simulink model "aerodymic_modules"  (R2023b)
settings: Solver=VariableStepAuto  StartTime=0.0  StopTime=simtime  MaxStep=0.00005  RelTol=1e-3
undefined symbols (not defined in the file): c_aero, c_drt, dpomega0, dpomega1, dpv1, dpv2, H_gen, H_WTR, k_a, k_aero, k_drt, lambda_opt, omega_0, omega_WTR_0, omega_WTR_n, p_avail, p_init, R_WTR, tau_init, Theta_0, Theta_vw2, Theta_w0, v_omega_1, v_w_0, v_w_min, v_w_n
settings Model: Creator=s183702  LastModifiedBy=marti

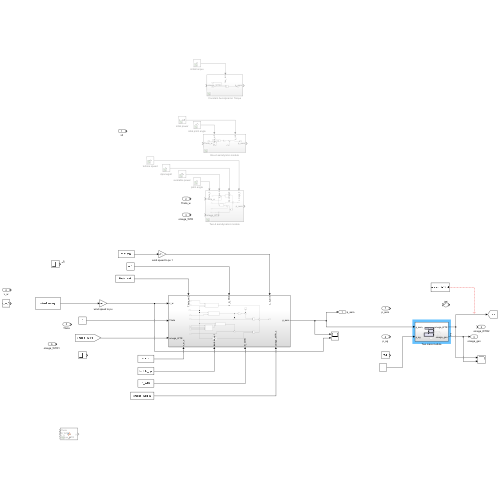
[thumbnail: Simulink's stored preview of the top-level diagram]
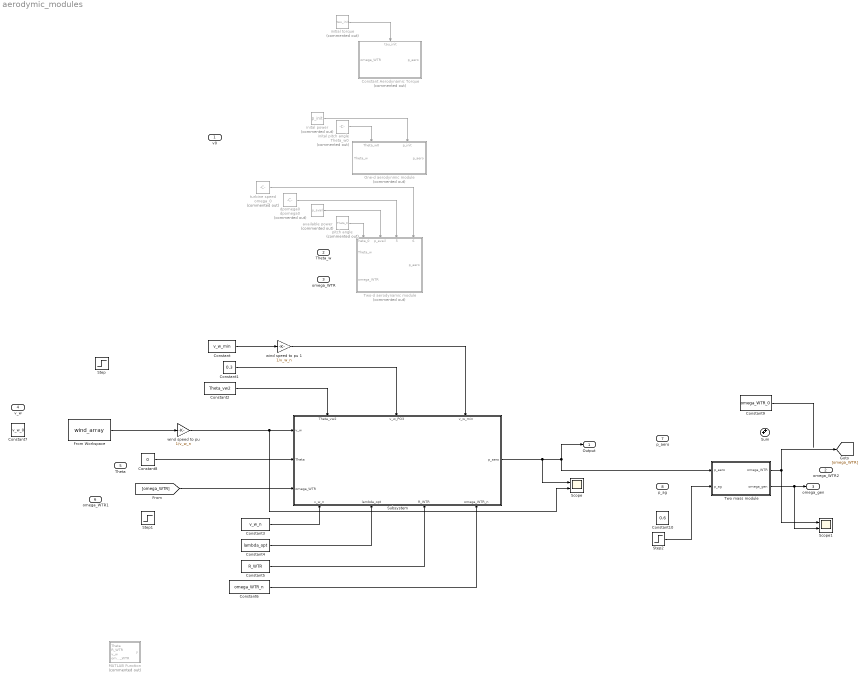
== system aerodymic_modules ==
  v0 : Inport
  Theta_w : Inport  Port=2
  omega_WTR : Inport  Port=3
  v_w : Inport  Port=4
  Theta : Inport  Port=5
  omega_WTR1 : Inport  Port=6
  p_aero : Inport  Port=7
  p_ag : Inport  Port=8
  Constant : Constant  Value=v_w_min
  Constant Aerodynamic Torque : Subsystem  Commented=on
      settings: PortSchema="{\"entries\":[{\"content\":{\"sides\":[{\"content\":{\"connectorIds\":[\"In1\"]},\"type\":\"ConnectorPlacement.EquallySpacedRectSide\",\"uuid\":\"8856b20c-a913-4b1f-bb06-3bfd5591729e\"},{\"content\":{\"connectorIds\":[\"Out1\"],\"side\":\"RIGHT\"},\"type\":\"ConnectorPlacement.EquallySpacedRectSide\",\"uuid\":\"d2cddd21-94c4-4346-9f93-c8cf69895e41\"},{\"content\":{\"connectorIds\":[\"In2\"],\"side\":\"TOP\"},\"type\":\"ConnectorPlacement.EquallySpacedRectSide\",\"uuid\":\"bedbe1d1-3c36-4165-aa7e-0fef857489e1\"},{\"content\":{\"side\":\"BOTTOM\"},\"type\":\"ConnectorPlacement.EquallySpacedRectSide\",\"uuid\":\"8fbc4b09-9296-41c8-ae54-d2fa1c44f1b6\"}]},\"type\":\"ConnectorPlacement.EquallySpacedConnector\",\"uuid\":\"9cd9660b-1bf9-4aa1-9147-9c9a71ae45e0\"}],\"packageUris\":[\"http://schema.mathworks.com/mf0/Connector/R2020b\"],\"version\":\"1.0\"}"
  Constant1 : Constant  Value=0.3
  Constant10 : Constant  Value=0.6
  Constant2 : Constant  Value=Theta_vw2
  Constant3 : Constant  Value=v_w_n
  Constant4 : Constant  Value=lambda_opt
  Constant5 : Constant  Value=R_WTR
  Constant6 : Constant  Value=omega_WTR_n
  Constant7 : Constant  Value=v_w_0
  Constant8 : Constant  Value=0
  Constant9 : Constant  Value=omega_WTR_0
  From Workspace : FromWorkspace  VariableName=wind_array
  MATLAB Function : MATLAB Function  Commented=on  TreatAsAtomicUnit=on
  One-d aerodynmic module : Subsystem  Commented=on
      settings: PortSchema="{\"entries\":[{\"content\":{\"sides\":[{\"content\":{\"connectorIds\":[\"In1\"]},\"type\":\"ConnectorPlacement.EquallySpacedRectSide\",\"uuid\":\"289bff7f-e2b1-4f4a-a280-3eccfab6ccfb\"},{\"content\":{\"connectorIds\":[\"Out1\"],\"side\":\"RIGHT\"},\"type\":\"ConnectorPlacement.EquallySpacedRectSide\",\"uuid\":\"ad352476-6e1f-4395-a3cf-73973636468c\"},{\"content\":{\"connectorIds\":[\"In2\",\"In3\"],\"side\":\"TOP\"},\"type\":\"ConnectorPlacement.EquallySpacedRectSide\",\"uuid\":\"0dc03381-ab12-4ca7-95d7-b6e9390f3624\"},{\"content\":{\"side\":\"BOTTOM\"},\"type\":\"ConnectorPlacement.EquallySpacedRectSide\",\"uuid\":\"0b978398-81f6-4235-820d-3640bddfbdb8\"}]},\"type\":\"ConnectorPlacement.EquallySpacedConnector\",\"uuid\":\"cacb7d17-2ea4-44c7-b4a3-963f0a31b934\"}],\"packageUris\":[\"http://schema.mathworks.com/mf0/Connector/R2020b\"],\"version\":\"1.0\"}"
  Scope : Scope  NumInputPorts=2
  Scope1 : Scope  NumInputPorts=2
  Step : Step  Time=11  Before=v_w_0  After=v_w_0+0.05  SampleTime=0
  Step1 : Step  Time=8  Before=omega_WTR_0  After=omega_WTR_0+0.1  SampleTime=0
  Step2 : Step  Time=20  Before=0.6  After=0.6  SampleTime=0
  Subsystem : Subsystem
      settings: PortSchema="{\"entries\":[{\"content\":{\"sides\":[{\"content\":{\"connectorIds\":[\"In1\",\"In2\",\"In3\"]},\"type\":\"ConnectorPlacement.EquallySpacedRectSide\",\"uuid\":\"ae3b79f5-547b-4d10-abca-a0aa9cd2564f\"},{\"content\":{\"connectorIds\":[\"Out1\"],\"side\":\"RIGHT\"},\"type\":\"ConnectorPlacement.EquallySpacedRectSide\",\"uuid\":\"c3c2b3cb-a75a-4372-91a9-47eb1a58d54f\"},{\"content\":{\"connectorIds\":[\"In4\",\"In5\",\"In6\"],\"side\":\"TOP\"},\"type\":\"ConnectorPlacement.EquallySpacedRectSide\",\"uuid\":\"49d081fd-d1d3-413c-affe-c564a0af719c\"},{\"content\":{\"connectorIds\":[\"In7\",\"In8\",\"In9\",\"In10\"],\"side\":\"BOTTOM\"},\"type\":\"ConnectorPlacement.EquallySpacedRectSide\",\"uuid\":\"c00a81a2-52c7-4daf-8b0c-a778841ec5d6\"}]},\"type\":\"ConnectorPlacement.EquallySpacedConnector\",\"uuid\":\"220248d6-ce4a-4e11-ab43-1d105a3d9686\"}],\"packageUris\":[\"http://schema.mathworks.com/mf0/Connector/R2020b\"],\"version\":\"1.0\"}"
  Sum : Sum  Inputs=++|
  Two mass module : Subsystem
  Two-d aerodynamic module : Subsystem  Commented=on
      settings: PortSchema="{\"entries\":[{\"content\":{\"sides\":[{\"content\":{\"connectorIds\":[\"In1\",\"In2\"]},\"type\":\"ConnectorPlacement.EquallySpacedRectSide\",\"uuid\":\"29aafb7d-ac63-4bda-a4d9-7691da9bab26\"},{\"content\":{\"connectorIds\":[\"Out1\"],\"side\":\"RIGHT\"},\"type\":\"ConnectorPlacement.EquallySpacedRectSide\",\"uuid\":\"d2e3e6f1-e433-4ce8-a4cd-da131dd7b9aa\"},{\"content\":{\"connectorIds\":[\"In3\",\"In4\",\"In5\",\"In6\"],\"side\":\"TOP\"},\"type\":\"ConnectorPlacement.EquallySpacedRectSide\",\"uuid\":\"d4b21252-afd5-4f00-9115-123c5cb74ac3\"},{\"content\":{\"side\":\"BOTTOM\"},\"type\":\"ConnectorPlacement.EquallySpacedRectSide\",\"uuid\":\"8ed30fa1-595f-4836-a19a-9de8ec421887\"}]},\"type\":\"ConnectorPlacement.EquallySpacedConnector\",\"uuid\":\"9c06a76b-7ab3-4f8d-9ed4-36342eae06f9\"}],\"packageUris\":[\"http://schema.mathworks.com/mf0/Connector/R2020b\"],\"version\":\"1.0\"}"
  available power : Constant  Commented=on  Value=p_avail
  dpomega0 : Constant  Commented=on  Value=dpomega0
  inital pitch angle : Constant  Commented=on  Value=Theta_w0
  inital power : Constant  Commented=on  Value=p_init
  initial torque : Constant  Commented=on  Value=tau_init
  pitch angle : Constant  Commented=on  Value=Theta_0
  turbine speed : Constant  Commented=on  Value=omega_0
  "wind speed to pu " : Gain  Gain=1/v_w_n
  wind speed to pu 1 : Gain  Gain=1/v_w_n
  Output : Outport  SignalName=p_aero
  omega_WTR2 : Outport  Port=2
  omega_gen : Outport  Port=3
  wires:
  initial torque/1 -> Constant Aerodynamic Torque/2(tau_init)
  inital pitch angle/1 -> One-d aerodynmic module/2(Theta_w0)
  inital power/1 -> One-d aerodynmic module/3(p_init)
  pitch angle/1 -> Two-d aerodynamic module/3(Theta_0)
  available power/1 -> Two-d aerodynamic module/4(p_avail)
  dpomega0/1 -> Two-d aerodynamic module/5(dpomega0)
  turbine speed/1 -> Two-d aerodynamic module/6(omega_0)
  Constant/1 -> wind speed to pu 1/1
  Constant1/1 -> Subsystem/5(v_w_PO3)
  From Workspace/1 -> "wind speed to pu "/1
  Constant2/1 -> Subsystem/4(Theta_vw2)
  Constant8/1 -> Subsystem/2(Theta)
  Constant3/1 -> Subsystem/7(v_w_n)
  Constant4/1 -> Subsystem/8(lambda_opt)
  Constant5/1 -> Subsystem/9(R_WTR)
  Constant6/1 -> Subsystem/10(omega_WTR_n)
  [omega_WTR] -> Subsystem/3(omega_WTR)
  wind speed to pu 1/1 -> Subsystem/6(v_w_min)
  Subsystem/1(p_aero) -> Scope/1, Two mass module/1(p_aero), Output/1
  Step2/1 -> Two mass module/2(p_ag)
  Two mass module/2(omega_gen) -> Scope1/2, omega_gen/1
  Constant9/1 -> ?
  Two mass module/1(omega_WTR) -> [omega_WTR], Scope1/1
  "wind speed to pu "/1 -> Scope/2, Subsystem/1(v_w)

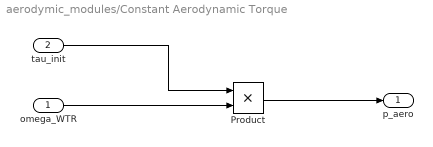
== system aerodymic_modules/Constant Aerodynamic Torque ==
  omega_WTR : Inport
  tau_init : Inport  Port=2
  Product : Product
  p_aero : Outport
  wires:
  omega_WTR/1 -> Product/2
  Product/1 -> p_aero/1
  tau_init/1 -> Product/1

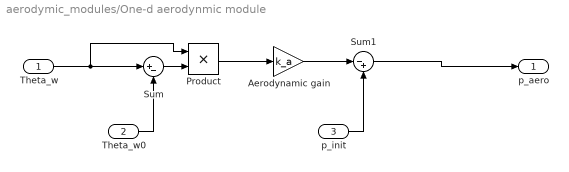
== system aerodymic_modules/One-d aerodynmic module ==
  Theta_w : Inport
  Theta_w0 : Inport  Port=2
  p_init : Inport  Port=3
  Aerodynamic gain : Gain  Gain=k_a
  Product : Product
  Sum : Sum  Inputs=|+-
  Sum1 : Sum  Inputs=|-+
  p_aero : Outport
  wires:
  Aerodynamic gain/1 -> Sum1/1
  Sum/1 -> Product/2
  Product/1 -> Aerodynamic gain/1
  Theta_w0/1 -> Sum/2
  p_init/1 -> Sum1/2
  Theta_w/1 -> Product/1, Sum/1
  Sum1/1 -> p_aero/1

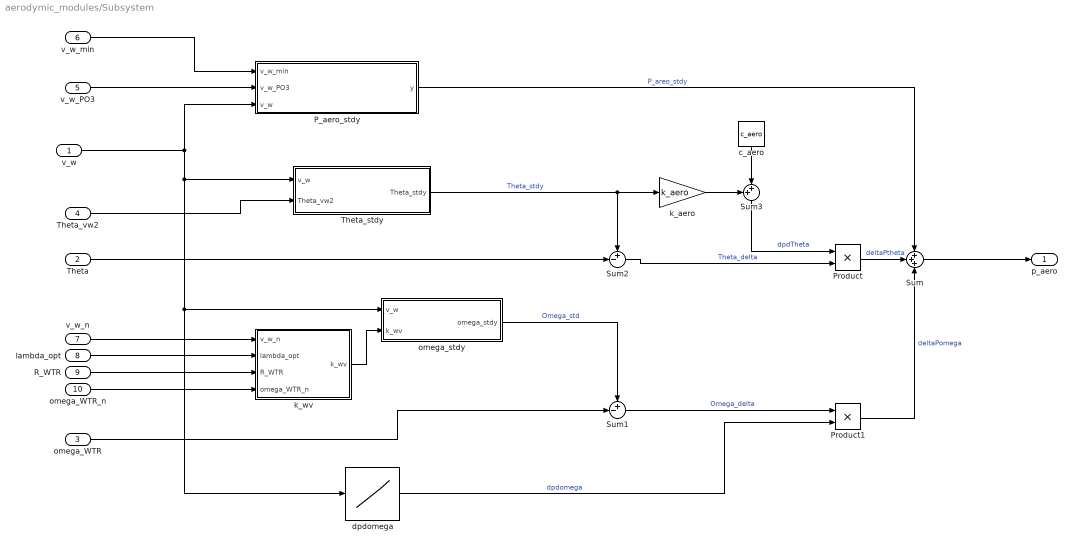
== system aerodymic_modules/Subsystem ==
  v_w : Inport
  Theta : Inport  Port=2
  omega_WTR : Inport  Port=3
  Theta_vw2 : Inport  Port=4
  v_w_PO3 : Inport  Port=5
  v_w_min : Inport  Port=6
  v_w_n : Inport  Port=7
  lambda_opt : Inport  Port=8
  R_WTR : Inport  Port=9
  omega_WTR_n : Inport  Port=10
  P_aero_stdy : MATLAB Function  TreatAsAtomicUnit=on
  Product : Product
  Product1 : Product
  Sum : Sum  Inputs=+++
  Sum1 : Sum  Inputs=+-|
  Sum2 : Sum  Inputs=+-|
  Sum3 : Sum  Inputs=++|
  Theta_stdy : MATLAB Function  TreatAsAtomicUnit=on
  c_aero : Constant  Value=c_aero
  dpdomega : Lookup_n-D  NumberOfTableDimensions=1  BreakpointsForDimension1=[0 v_omega_1 1 2]  BreakpointsForDimension3=[5, 7]  Table="[dpomega1 dpomega1  dpv1 dpv2]"  InternalRulePriority=Speed  RndMeth=Simplest
  k_aero : Gain  Gain=k_aero
  k_wv : MATLAB Function  TreatAsAtomicUnit=on
  omega_stdy : MATLAB Function  TreatAsAtomicUnit=on
  p_aero : Outport
  wires:
  k_aero/1 -> Sum3/1
  Sum3/1 -> Product/1  "dpdTheta"
  c_aero/1 -> Sum3/2
  dpdomega/1 -> Product1/2  "dpdomega"
  Product/1 -> Sum/2  "deltaPtheta"
  omega_WTR_n/1 -> k_wv/4(omega_WTR_n)
  Product1/1 -> Sum/3  "deltaPomega"
  Theta_stdy/1(Theta_stdy) -> k_aero/1, Sum2/1  "Theta_stdy"
  P_aero_stdy/1(y) -> Sum/1  "P_areo_stdy"
  Theta_vw2/1 -> Theta_stdy/2(Theta_vw2)
  R_WTR/1 -> k_wv/3(R_WTR)
  k_wv/1(k_wv) -> omega_stdy/2(k_wv)
  v_w_min/1 -> P_aero_stdy/1(v_w_min)
  Sum1/1 -> Product1/1  "Omega_delta"
  v_w_n/1 -> k_wv/1(v_w_n)
  Sum2/1 -> Product/2  "Theta_delta"
  omega_stdy/1(omega_stdy) -> Sum1/1  "Omega_std"
  lambda_opt/1 -> k_wv/2(lambda_opt)
  v_w/1 -> P_aero_stdy/3(v_w), Theta_stdy/1(v_w), dpdomega/1, omega_stdy/1(v_w)
  omega_WTR/1 -> Sum1/2
  Theta/1 -> Sum2/2
  v_w_PO3/1 -> P_aero_stdy/2(v_w_PO3)
  Sum/1 -> p_aero/1

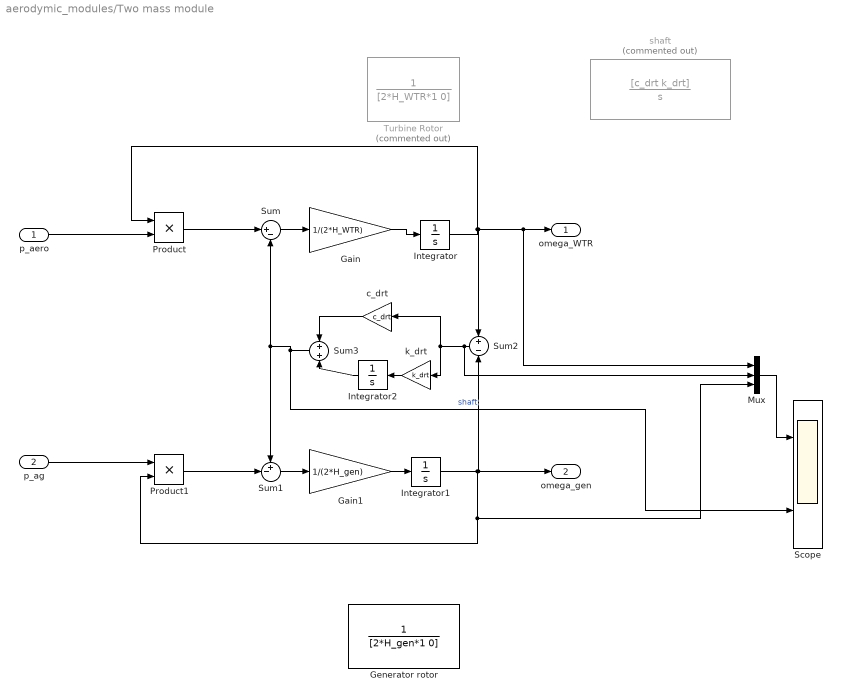
== system aerodymic_modules/Two mass module ==
  p_aero : Inport
  p_ag : Inport  Port=2
  Gain : Gain  Gain=1/(2*H_WTR)
  Gain1 : Gain  Gain=1/(2*H_gen)
  Generator rotor : TransferFcn  Denominator=[2*H_gen*1 0]
  Integrator : Integrator  InitialCondition=omega_WTR_0
  Integrator1 : Integrator  InitialCondition=omega_WTR_0
  Integrator2 : Integrator
  Mux : Mux  Inputs=3
  Product : Product
  Product1 : Product
  Scope : Scope  NumInputPorts=2
  Sum : Sum  Inputs=|+-
  Sum1 : Sum  Inputs=+-|
  Sum2 : Sum  Inputs=+|-
  Sum3 : Sum  Inputs=+|+
  Turbine Rotor : TransferFcn  Commented=on  Denominator=[2*H_WTR*1 0]
  c_drt : Gain  Gain=c_drt
  k_drt : Gain  Gain=k_drt
  shaft : TransferFcn  Commented=on  Numerator=[c_drt k_drt]  Denominator=[1 0]
  omega_WTR : Outport
  omega_gen : Outport  Port=2
  wires:
  Product1/1 -> Sum1/2
  Integrator1/1 -> omega_gen/1, Sum2/2, Mux/3, Product1/2
  Sum3/1 -> Sum1/1, Sum/2, Scope/2  "shaft"
  Integrator/1 -> Mux/1, omega_WTR/1, Sum2/1, Product/1
  Sum/1 -> Gain/1
  p_ag/1 -> Product1/1
  p_aero/1 -> Product/2
  Product/1 -> Sum/1
  Gain/1 -> Integrator/1
  Gain1/1 -> Integrator1/1
  Sum1/1 -> Gain1/1
  Integrator2/1 -> Sum3/2
  c_drt/1 -> Sum3/1
  Sum2/1 -> Mux/2, k_drt/1, c_drt/1
  k_drt/1 -> Integrator2/1
  Mux/1 -> Scope/1

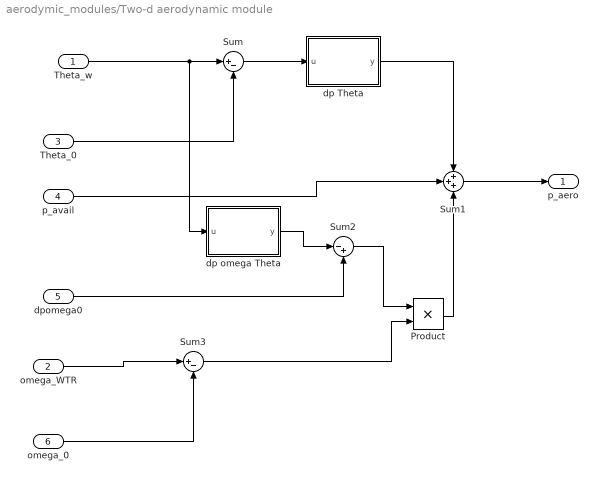
== system aerodymic_modules/Two-d aerodynamic module ==
  Theta_w : Inport
  omega_WTR : Inport  Port=2
  Theta_0 : Inport  Port=3
  p_avail : Inport  Port=4
  dpomega0 : Inport  Port=5
  omega_0 : Inport  Port=6
  Product : Product
  Sum : Sum  Inputs=|+-
  Sum1 : Sum  Inputs=+++
  Sum2 : Sum  Inputs=|-+
  Sum3 : Sum  Inputs=|+-
  dp Theta : MATLAB Function  TreatAsAtomicUnit=on
  dp omega Theta : MATLAB Function  TreatAsAtomicUnit=on
  p_aero : Outport
  wires:
  Theta_w/1 -> dp omega Theta/1(u), Sum/1
  Sum2/1 -> Product/1
  Product/1 -> Sum1/3
  dp omega Theta/1(y) -> Sum2/1
  Sum/1 -> dp Theta/1(u)
  dp Theta/1(y) -> Sum1/1
  Sum3/1 -> Product/2
  omega_WTR/1 -> Sum3/1
  Sum1/1 -> p_aero/1
  Theta_0/1 -> Sum/2
  omega_0/1 -> Sum3/2
  p_avail/1 -> Sum1/2
  dpomega0/1 -> Sum2/2

== matlab function aerodymic_modules/Two-d aerodynamic module/dp omega Theta ==
  data: u input; y output
function y = fcn(u)

y = u;

== matlab function aerodymic_modules/Two-d aerodynamic module/dp Theta ==
  data: u input; y output
function y = fcn(u)

y = u;

== matlab function aerodymic_modules/Subsystem/P_aero_stdy ==
  data: v_w_min input; v_w_PO3 input; v_w input; y output
function y = p_aero_stdy(v_w_min,v_w_PO3,v_w)
x=0;

if (v_w_min <= v_w) && (v_w < v_w_PO3)
         x = 0.3/(v_w_PO3^3)*(v_w^3);
elseif (v_w_PO3 <= v_w) && (v_w < 1)
        x = 1+(v_w-1)*0.7/(1-v_w_PO3);
elseif 1 <= v_w
        x = 1;
end
y = x;

== matlab function aerodymic_modules/Subsystem/Theta_stdy ==
  data: v_w input; Theta_stdy output; Theta_vw2 input
function Theta_stdy = Theta_stdy(v_w,Theta_vw2)


if v_w < 1
    x = 0;
else
    x = Theta_vw2*4/3*(1-1/v_w^2);
end

Theta_stdy = x;

== matlab function aerodymic_modules/Subsystem/omega_stdy ==
  data: v_w input; omega_stdy output; k_wv input
function omega_stdy = omega_stdy(v_w,k_wv)

omega_stdy = v_w*k_wv;

== matlab function aerodymic_modules/Subsystem/k_wv ==
  data: v_w_n input; k_wv output; lambda_opt input; R_WTR input; omega_WTR_n input
function k_wv = k_wv(v_w_n,lambda_opt,R_WTR,omega_WTR_n)

k_wv = lambda_opt*v_w_n/(R_WTR*omega_WTR_n);

== matlab function aerodymic_modules/MATLAB Function ==
  data: Theta input; y output; R_WTR input; v_w input; omega_WTR input
function y = c_p(Theta,R_WTR,v_w,omega_WTR)

    lambda    
    c = [0.645 116 0.4 5 21 0.00912 0.08 0.035 0.001];
    a = (-c(4)-c(3)*(2.5+Theta)+c(2)*1/(lambda+c(7)*(2.5+Theta))-c(8)/(lambda+(2.5+Theta)^3));
    exponent = c(5)*1/(lambda+c(7)*(2.5+Theta))-c(8)/(lambda+(2.5+Theta)^3);
    x = c(1)*(c(6)*lambda+a/exp(exponent))+c(9)*lambda;

y = ;
